simulink model "HGvwab"  (R2020b)
settings: Solver=VariableStepAuto  StartTime=0.0  StopTime=T  MaxStep=MaxStep  RelTol=RelTol  EnableMultiTasking=on
values from neighbouring files (symbols this model uses):
  c = -55    [main.m]
  d = 4    [main.m]
  delay_m = 0    [main.m]
  Iext = 10    [main.m]
  J = 10    [main.m]
  ll = 4    [main.m]
  rule = 1    [main.m]
  T = 30    [main.m]
  x0 = [-55;-6;a;b]    [main.m]
  zHat0 = compute_z(xHat0,Iext)    [main.m]
undefined symbols (not defined in the file or in its folder): C_syst, compute_cond_inv, compute_cond_inv_z, compute_x, compute_z, D_syst, f_syst, g_syst
libraries: simulink x6
settings Model: Creator=pmbernar  LastModifiedBy=Pauline
settings DataIOCC: LimitDataPoints=on  ReturnWorkspaceOutputs=off
settings OptimizationCC: LifeSpan=inf
settings DebuggingCC: AllowSymbolicDim=off  PregeneratedLibrarySubsystemCodeDiagnostic=none  SFUnexpectedBacktrackingDiag=warning  SFNoUnconditionalDefaultTransitionDiag=warning  SFExecutionAtInitializationDiag=none  ArithmeticOperatorsInVariantConditions=warning
settings ModelReferenceCC: PropagateSignalLabelsOutOfModel=off
settings SFSimCC: SimUseLocalCustomCode=off  CustomCodeUndefinedFunction=UseInterfaceOnly
settings RTWCC: RTWUseLocalCustomCode=off
settings CodeAppCC: StateflowObjectComments=on
settings GRTTargetCC: TargetLangStandard=C89/C90 (ANSI)
settings ConfigComp: CovMetricSettings=dw  CovSaveCumulativeToWorkspaceVar=on  CovSaveSingleToWorkspaceVar=on  CovExternalEMLEnable=off

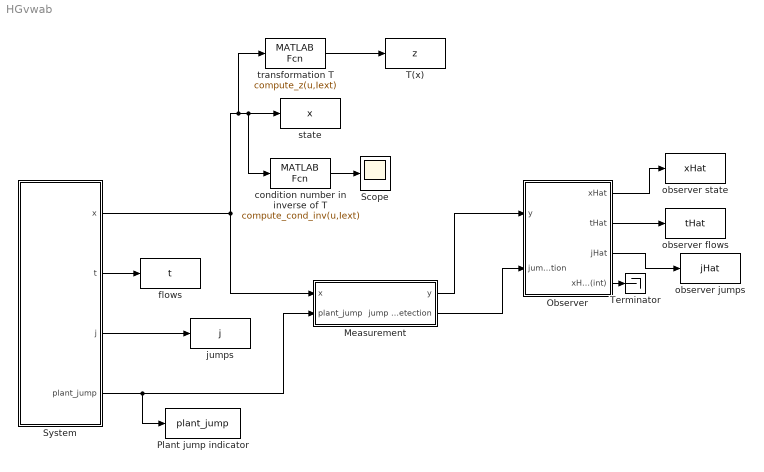
== system HGvwab ==
  Measurement : Subsystem  TreatAsAtomicUnit=on
  Observer : Subsystem  LoadFcn=set_param(gcb,'LinkStatus','none')
      settings: CopyFcn=|
      | set_param(gcb,'LinkStatus','none'),
      | set_param(gcs, 'MaxStep', 'MaxStep', 'RelTol', 'RelTol','Stop time', 'T')
  Plant jump indicator : ToWorkspace  VariableName=plant_jump  SampleTime=-1
  Scope : Scope
  System : Subsystem  LoadFcn=set_param(gcb,'LinkStatus','none')
      settings: CopyFcn=set_param(gcb,'LinkStatus','none')
      mask Display:
      | %image(imread('Hcalneg.jpg'))
      | %plot([5 20 20 5 5],[5 5 20 20 5])
      | %text(8,13,'HyEq_mdl')
      | color('white')
      | port_label('output', 1, 'x')
      | port_label('output', 2, 't')
      | port_label('output', 3, 'j')
  "T(x) " : ToWorkspace  VariableName=z  SampleTime=-1
  Terminator : Terminator
  "condition number in inverse of T " : MATLABFcn  MATLABFcn=compute_cond_inv(u,Iext)
  flows : ToWorkspace  VariableName=t  SampleTime=-1
  jumps : ToWorkspace  VariableName=j  SampleTime=-1
  observer flows : ToWorkspace  VariableName=tHat  SampleTime=-1
  observer jumps : ToWorkspace  VariableName=jHat  SampleTime=-1
  observer state : ToWorkspace  VariableName=xHat  SampleTime=-1
  state : ToWorkspace  VariableName=x  SampleTime=-1
  transformation T : MATLABFcn  MATLABFcn=compute_z(u,Iext)
  wires:
  System/2(t) -> flows/1
  System/3(j) -> jumps/1
  Measurement/1(y) -> Observer/1(y)
  Observer/1(xHat) -> observer state/1
  Observer/2(tHat) -> observer flows/1
  Observer/3(jHat) -> observer jumps/1
  System/1(x) -> Measurement/1(x), transformation T/1, "condition number in inverse of T "/1, state/1
  transformation T/1 -> "T(x) "/1
  "condition number in inverse of T "/1 -> Scope/1
  Observer/4(xHat-(int)) -> Terminator/1
  System/4(plant_jump) -> Plant jump indicator/1, Measurement/2(plant_jump)
  Measurement/2(" jump detection") -> Observer/2(jump detection)

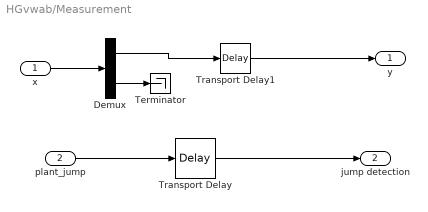
== system HGvwab/Measurement ==
  x : Inport
  plant_jump : Inport  Port=2
  Demux : Demux  Outputs=2
  Terminator : Terminator
  Transport Delay : TransportDelay  DelayTime=delay_m
  Transport Delay1 : TransportDelay  DelayTime=delay_m  InitialOutput=delay_m
  y : Outport  VectorParamsAs1DForOutWhenUnconnected=off
  " jump detection" : Outport  Port=2  VectorParamsAs1DForOutWhenUnconnected=off
  wires:
  x/1 -> Demux/1
  Transport Delay1/1 -> y/1
  Demux/1 -> Transport Delay1/1
  Demux/2 -> Terminator/1
  plant_jump/1 -> Transport Delay/1
  Transport Delay/1 -> " jump detection"/1

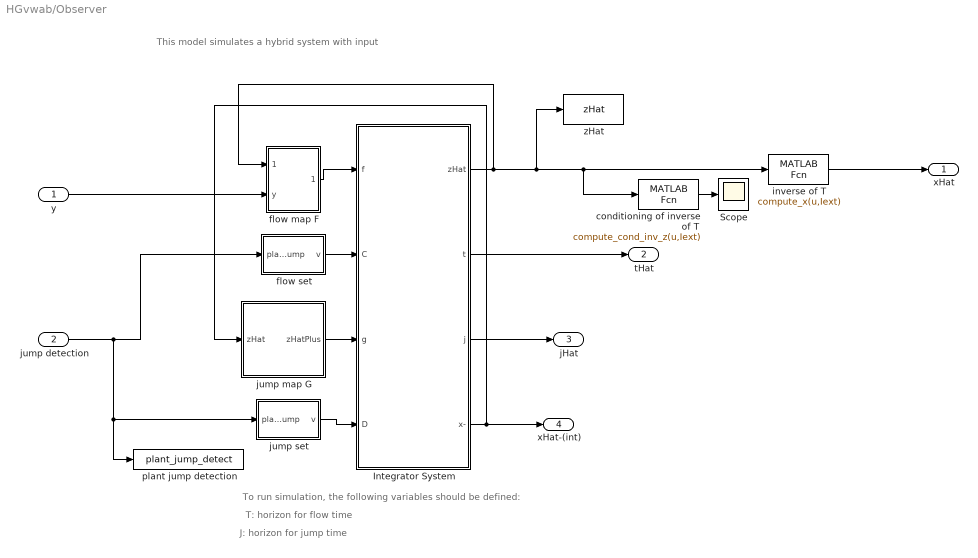
== system HGvwab/Observer ==
  note: J: horizon for jump time
  note: T: horizon for flow time
  note: To run simulation, the following variables should be defined:
  note: This model simulates a hybrid system with input
  y : Inport
  jump detection : Inport  Port=2
  Integrator System : Subsystem  Priority=2  mask(Hybrid Integrator){T=T, J=J, x0=zHat0}
      mask prompts: T "Flow Horizon"; J "Jump Horizon"; x0 "Initial Condition"
      mask help:
      | This block integrates the state of the hybrid system defined by the flow map f (first input), the flow set C (second input), the jump map g (third input) and the jump set D (fourth input).
      | Starting from the initial condition x0 (last mask parameter), the system's state x evolves continuously within the set C, according to f(x,u), but is also subject to jumps within D, according to g(x,u).
      | The block also stops the simulation when the time t is greater than the flow horizon T (first mask parameter), or when the number of jumps j is greater than the jump horizon J (second mask parameter).
      | The outputs of the blocks are respectively x(t), t, j, x(t-).
      mask Help:
      | This block integrates the state of the hybrid system defined by the flow map f (first input), the flow set C (second input), the jump map g (third input) and the jump set D (fourth input).
      | <br>
      | Starting from the initial condition x0 (last mask parameter), the system's state x evolves continuously within the set C, according to f(x,u), but is also subject to jumps within D, according to g(x,u).
      | <br>
      | The block also stops the simulation when the time t is greater than the flow horizon T (first mask parameter), or when the number of jumps j is greater than the jump horizon J (second mask parameter).
      | <br>
      | The outputs of the blocks are respectively x(t), t, j, x(t-).
      | <br>
      | You can right click on the block and "Look under mask" to see what's inside the block.
      | Finally, refer to the manual (HybridSimulator_vXX.pdf) for more detailed information on how this hybrid simulator works.
  Scope : Scope
  conditioning of inverse of T : MATLABFcn  MATLABFcn=compute_cond_inv_z(u,Iext)
  flow map F : MATLAB Function  TreatAsAtomicUnit=on
  "flow set " : MATLAB Function  TreatAsAtomicUnit=on
  inverse of T : MATLABFcn  MATLABFcn=compute_x(u,Iext)
  jump map G : MATLAB Function  Priority=2  TreatAsAtomicUnit=on
  "jump set " : MATLAB Function  TreatAsAtomicUnit=on
  plant jump detection : ToWorkspace  VariableName=plant_jump_detect  SampleTime=-1
  zHat : ToWorkspace  VariableName=zHat  SampleTime=-1
  xHat : Outport  VectorParamsAs1DForOutWhenUnconnected=off
  tHat : Outport  Port=2  VectorParamsAs1DForOutWhenUnconnected=off
  jHat : Outport  Port=3  VectorParamsAs1DForOutWhenUnconnected=off
  xHat-(int) : Outport  Port=4  VectorParamsAs1DForOutWhenUnconnected=off
  wires:
  jump map G/1(zHatPlus) -> Integrator System/3(g)
  "jump set "/1(v) -> Integrator System/4(D)
  y/1 -> flow map F/2(y)
  Integrator System/3(j) -> jHat/1
  Integrator System/2(t) -> tHat/1
  "flow set "/1(v) -> Integrator System/2(C)
  Integrator System/1(zHat) -> zHat/1, conditioning of inverse of T/1, inverse of T/1, flow map F/1(zHat)
  Integrator System/4(x-) -> jump map G/1(zHat), xHat-(int)/1
  flow map F/1(zHatdot) -> Integrator System/1(f)
  inverse of T/1 -> xHat/1
  conditioning of inverse of T/1 -> Scope/1
  jump detection/1 -> "flow set "/1(plant_jump), "jump set "/1(plant_jump), plant jump detection/1

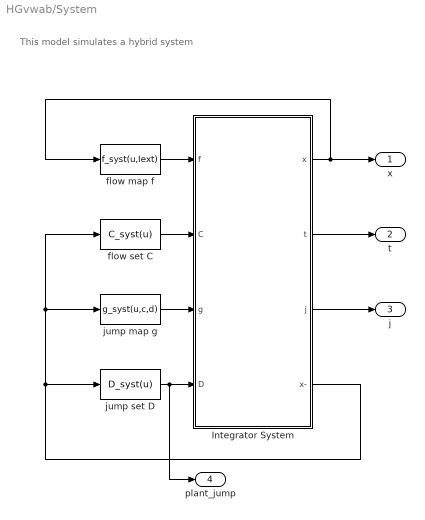
== system HGvwab/System ==
  note: This model simulates a hybrid system
  Integrator System : Subsystem  Priority=2  mask(Hybrid Integrator){T=T, J=J, x0=x0}
      mask prompts: T "Flow Horizon"; J "Jump Horizon"; x0 "Initial Condition"
      mask help:
      | This block integrates the state of the hybrid system defined by the flow map f (first input), the flow set C (second input), the jump map g (third input) and the jump set D (fourth input).
      | Starting from the initial condition x0 (last mask parameter), the system's state x evolves continuously within the set C, according to f(x,u), but is also subject to jumps within D, according to g(x,u).
      | The block also stops the simulation when the time t is greater than the flow horizon T (first mask parameter), or when the number of jumps j is greater than the jump horizon J (second mask parameter).
      | The outputs of the blocks are respectively x(t), t, j, x(t-).
      mask Help:
      | This block integrates the state of the hybrid system defined by the flow map f (first input), the flow set C (second input), the jump map g (third input) and the jump set D (fourth input).
      | <br>
      | Starting from the initial condition x0 (last mask parameter), the system's state x evolves continuously within the set C, according to f(x,u), but is also subject to jumps within D, according to g(x,u).
      | <br>
      | The block also stops the simulation when the time t is greater than the flow horizon T (first mask parameter), or when the number of jumps j is greater than the jump horizon J (second mask parameter).
      | <br>
      | The outputs of the blocks are respectively x(t), t, j, x(t-).
      | <br>
      | You can right click on the block and "Look under mask" to see what's inside the block.
      | Finally, refer to the manual (HybridSimulator_vXX.pdf) for more detailed information on how this hybrid simulator works.
  flow map f : MATLABFcn  MATLABFcn=f_syst(u,Iext)
  flow set C : MATLABFcn  MATLABFcn=C_syst(u)
  jump map g : MATLABFcn  MATLABFcn=g_syst(u,c,d)
  jump set D : MATLABFcn  MATLABFcn=D_syst(u)
  x : Outport  VectorParamsAs1DForOutWhenUnconnected=off
  t : Outport  Port=2  VectorParamsAs1DForOutWhenUnconnected=off
  j : Outport  Port=3  VectorParamsAs1DForOutWhenUnconnected=off
  plant_jump : Outport  Port=4
  wires:
  jump map g/1 -> Integrator System/3(g)
  jump set D/1 -> plant_jump/1, Integrator System/4(D)
  Integrator System/3(j) -> j/1
  Integrator System/2(t) -> t/1
  flow set C/1 -> Integrator System/2(C)
  Integrator System/1(x) -> flow map f/1, x/1
  Integrator System/4(x-) -> flow set C/1, jump map g/1, jump set D/1
  flow map f/1 -> Integrator System/1(f)

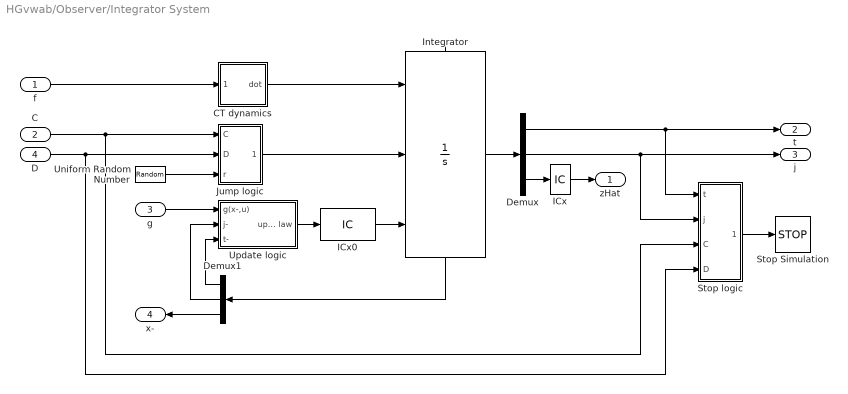
== system HGvwab/Observer/Integrator System ==
  f : Inport
  C : Inport  Port=2
  g : Inport  Port=3
  D : Inport  Port=4
  CT dynamics : Subsystem
  Demux : Demux  Outputs=[1 1 -1]
  Demux1 : Demux  Outputs=[1 1 -1]
  ICx : InitialCondition  Value=x0
  ICx0 : InitialCondition  Value=[0; 0; x0(:)]
  Integrator : Integrator  ExternalReset=level hold  InitialConditionSource=external  ShowStatePort=on  ZeroCross=off
  Jump logic : Subsystem
  Stop Simulation : Stop
  Stop logic : Subsystem
  Uniform Random Number : UniformRandomNumber  Minimum=0  Seed=abs(floor(100*rand))  SampleTime=0
  Update logic : Subsystem
  zHat : Outport  VectorParamsAs1DForOutWhenUnconnected=off
  t : Outport  Port=2  VectorParamsAs1DForOutWhenUnconnected=off
  j : Outport  Port=3  VectorParamsAs1DForOutWhenUnconnected=off
  x- : Outport  Port=4  VectorParamsAs1DForOutWhenUnconnected=off
  wires:
  ICx0/1 -> Integrator/3
  ICx/1 -> zHat/1
  Demux/3 -> ICx/1
  Integrator/State -> Demux1/1
  Demux/2 -> j/1, Stop logic/2(j)
  Demux/1 -> t/1, Stop logic/1(t)
  Update logic/1(update law) -> ICx0/1
  CT dynamics/1(dot) -> Integrator/1
  Stop logic/1(stop) -> Stop Simulation/1
  Integrator/1 -> Demux/1
  C/1 -> Stop logic/3(C), Jump logic/1(C)
  D/1 -> Stop logic/4(D), Jump logic/2(D)
  f/1 -> CT dynamics/1(f(x,u))
  Demux1/3 -> x-/1
  Jump logic/1(jump) -> Integrator/2
  Uniform Random Number/1 -> Jump logic/3(r)
  g/1 -> Update logic/1(g(x-,u))
  Demux1/1 -> Update logic/3(t-)
  Demux1/2 -> Update logic/2(j-)

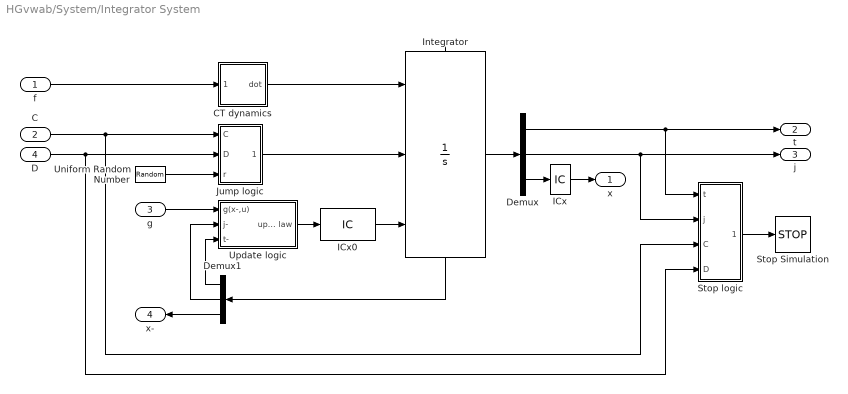
== system HGvwab/System/Integrator System ==
  f : Inport
  C : Inport  Port=2
  g : Inport  Port=3
  D : Inport  Port=4
  CT dynamics : Subsystem
  Demux : Demux  Outputs=[1 1 -1]
  Demux1 : Demux  Outputs=[1 1 -1]
  ICx : InitialCondition  Value=x0
  ICx0 : InitialCondition  Value=[0; 0; x0(:)]
  Integrator : Integrator  ExternalReset=level hold  InitialConditionSource=external  ShowStatePort=on  ZeroCross=off
  Jump logic : Subsystem
  Stop Simulation : Stop
  Stop logic : Subsystem
  Uniform Random Number : UniformRandomNumber  Minimum=0  Seed=abs(floor(100*rand))  SampleTime=0
  Update logic : Subsystem
  x : Outport  VectorParamsAs1DForOutWhenUnconnected=off
  t : Outport  Port=2  VectorParamsAs1DForOutWhenUnconnected=off
  j : Outport  Port=3  VectorParamsAs1DForOutWhenUnconnected=off
  x- : Outport  Port=4  VectorParamsAs1DForOutWhenUnconnected=off
  wires:
  ICx0/1 -> Integrator/3
  ICx/1 -> x/1
  Demux/3 -> ICx/1
  Integrator/State -> Demux1/1
  Demux/2 -> j/1, Stop logic/2(j)
  Demux/1 -> t/1, Stop logic/1(t)
  Update logic/1(update law) -> ICx0/1
  CT dynamics/1(dot) -> Integrator/1
  Stop logic/1(stop) -> Stop Simulation/1
  Integrator/1 -> Demux/1
  C/1 -> Stop logic/3(C), Jump logic/1(C)
  D/1 -> Stop logic/4(D), Jump logic/2(D)
  f/1 -> CT dynamics/1(f(x,u))
  Demux1/3 -> x-/1
  Jump logic/1(jump) -> Integrator/2
  Uniform Random Number/1 -> Jump logic/3(r)
  g/1 -> Update logic/1(g(x-,u))
  Demux1/1 -> Update logic/3(t-)
  Demux1/2 -> Update logic/2(j-)

== system HGvwab/Observer/Integrator System/CT dynamics ==
  f(x,u) : Inport
  Flows : Constant
  Jumps : Constant  Value=0
  Mux : Mux  Inputs=[1 1 -1]
  dot : Outport  VectorParamsAs1DForOutWhenUnconnected=off
  wires:
  Jumps/1 -> Mux/2
  Flows/1 -> Mux/1
  Mux/1 -> dot/1
  f(x,u)/1 -> Mux/3

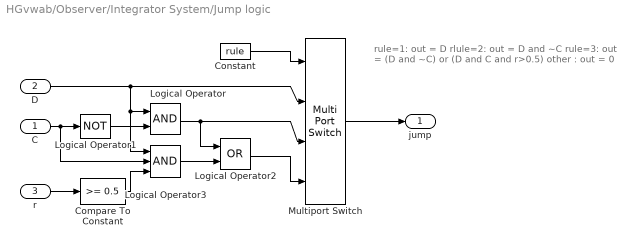
== system HGvwab/Observer/Integrator System/Jump logic ==
  note: rule=1:  out = D
      | rlule=2: out = D and ~C
      | rule=3:  out = (D and ~C)  or (D and C and r>0.5)
      | other :  out = 0
  C : Inport
  D : Inport  Port=2
  r : Inport  Port=3
  Compare To Constant : simulink/Logic and Bit Operations/Compare To Constant  relop=>=  const=0.5  OutDataTypeStr=uint8
  Constant : Constant  Value=rule
  Logical Operator : Logic  AllPortsSameDT=off  OutDataTypeStr=boolean
  Logical Operator1 : Logic  Operator=NOT  Inputs=1  AllPortsSameDT=off  OutDataTypeStr=boolean
  Logical Operator2 : Logic  Operator=OR  AllPortsSameDT=off  OutDataTypeStr=boolean
  Logical Operator3 : Logic  Inputs=3  AllPortsSameDT=off  OutDataTypeStr=boolean
  Multiport Switch : MultiPortSwitch
  jump : Outport  VectorParamsAs1DForOutWhenUnconnected=off
  wires:
  Constant/1 -> Multiport Switch/1
  D/1 -> Logical Operator3/1, Logical Operator/1, Multiport Switch/2
  r/1 -> Compare To Constant/1
  C/1 -> Logical Operator3/2, Logical Operator1/1
  Logical Operator1/1 -> Logical Operator/2
  Logical Operator/1 -> Multiport Switch/3, Logical Operator2/1
  Logical Operator2/1 -> Multiport Switch/4
  Multiport Switch/1 -> jump/1
  Compare To Constant/1 -> Logical Operator3/3
  Logical Operator3/1 -> Logical Operator2/2

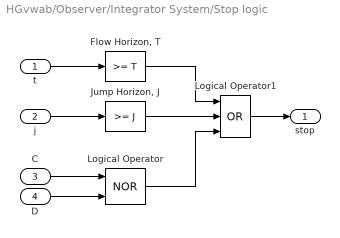
== system HGvwab/Observer/Integrator System/Stop logic ==
  t : Inport
  j : Inport  Port=2
  C : Inport  Port=3
  D : Inport  Port=4
  "Flow Horizon, T" : simulink/Logic and Bit Operations/Compare To Constant  relop=>=  const=T  OutDataTypeStr=uint8  ZeroCross=off
  "Jump Horizon, J" : simulink/Logic and Bit Operations/Compare To Constant  relop=>=  const=J  OutDataTypeStr=uint8  ZeroCross=off
  Logical Operator : Logic  Operator=NOR  AllPortsSameDT=off  OutDataTypeStr=boolean
  Logical Operator1 : Logic  Operator=OR  Inputs=3  AllPortsSameDT=off  OutDataTypeStr=boolean
  stop : Outport  VectorParamsAs1DForOutWhenUnconnected=off
  wires:
  "Flow Horizon, T"/1 -> Logical Operator1/1
  "Jump Horizon, J"/1 -> Logical Operator1/2
  Logical Operator/1 -> Logical Operator1/3
  D/1 -> Logical Operator/2
  t/1 -> "Flow Horizon, T"/1
  j/1 -> "Jump Horizon, J"/1
  C/1 -> Logical Operator/1
  Logical Operator1/1 -> stop/1

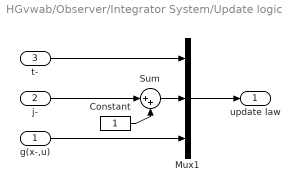
== system HGvwab/Observer/Integrator System/Update logic ==
  g(x-,u) : Inport
  j- : Inport  Port=2
  t- : Inport  Port=3
  Constant : Constant
  Mux1 : Mux  Inputs=[1 1 -1]
  Sum : Sum  Inputs=|++
  update law : Outport  VectorParamsAs1DForOutWhenUnconnected=off
  wires:
  Sum/1 -> Mux1/2
  Mux1/1 -> update law/1
  j-/1 -> Sum/1
  g(x-,u)/1 -> Mux1/3
  t-/1 -> Mux1/1
  Constant/1 -> Sum/2

== system HGvwab/System/Integrator System/CT dynamics ==
  f(x,u) : Inport
  Flows : Constant
  Jumps : Constant  Value=0
  Mux : Mux  Inputs=[1 1 -1]
  dot : Outport  VectorParamsAs1DForOutWhenUnconnected=off
  wires:
  Jumps/1 -> Mux/2
  Flows/1 -> Mux/1
  Mux/1 -> dot/1
  f(x,u)/1 -> Mux/3

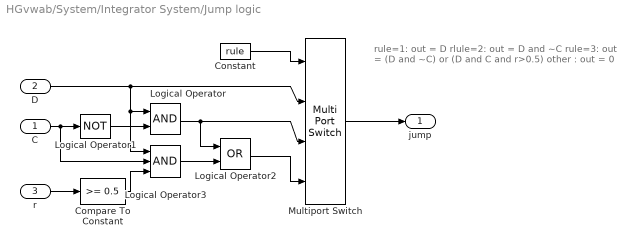
== system HGvwab/System/Integrator System/Jump logic ==
  note: rule=1:  out = D
      | rlule=2: out = D and ~C
      | rule=3:  out = (D and ~C)  or (D and C and r>0.5)
      | other :  out = 0
  C : Inport
  D : Inport  Port=2
  r : Inport  Port=3
  Compare To Constant : simulink/Logic and Bit Operations/Compare To Constant  relop=>=  const=0.5  OutDataTypeStr=uint8
  Constant : Constant  Value=rule
  Logical Operator : Logic  AllPortsSameDT=off  OutDataTypeStr=boolean
  Logical Operator1 : Logic  Operator=NOT  Inputs=1  AllPortsSameDT=off  OutDataTypeStr=boolean
  Logical Operator2 : Logic  Operator=OR  AllPortsSameDT=off  OutDataTypeStr=boolean
  Logical Operator3 : Logic  Inputs=3  AllPortsSameDT=off  OutDataTypeStr=boolean
  Multiport Switch : MultiPortSwitch
  jump : Outport  VectorParamsAs1DForOutWhenUnconnected=off
  wires:
  Constant/1 -> Multiport Switch/1
  D/1 -> Logical Operator3/1, Logical Operator/1, Multiport Switch/2
  r/1 -> Compare To Constant/1
  C/1 -> Logical Operator3/2, Logical Operator1/1
  Logical Operator1/1 -> Logical Operator/2
  Logical Operator/1 -> Multiport Switch/3, Logical Operator2/1
  Logical Operator2/1 -> Multiport Switch/4
  Multiport Switch/1 -> jump/1
  Compare To Constant/1 -> Logical Operator3/3
  Logical Operator3/1 -> Logical Operator2/2

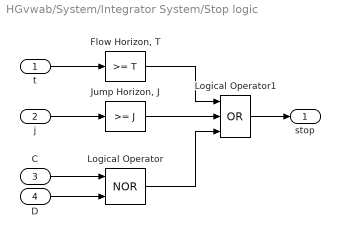
== system HGvwab/System/Integrator System/Stop logic ==
  t : Inport
  j : Inport  Port=2
  C : Inport  Port=3
  D : Inport  Port=4
  "Flow Horizon, T" : simulink/Logic and Bit Operations/Compare To Constant  relop=>=  const=T  OutDataTypeStr=uint8  ZeroCross=off
  "Jump Horizon, J" : simulink/Logic and Bit Operations/Compare To Constant  relop=>=  const=J  OutDataTypeStr=uint8  ZeroCross=off
  Logical Operator : Logic  Operator=NOR  AllPortsSameDT=off  OutDataTypeStr=boolean
  Logical Operator1 : Logic  Operator=OR  Inputs=3  AllPortsSameDT=off  OutDataTypeStr=boolean
  stop : Outport  VectorParamsAs1DForOutWhenUnconnected=off
  wires:
  "Flow Horizon, T"/1 -> Logical Operator1/1
  "Jump Horizon, J"/1 -> Logical Operator1/2
  Logical Operator/1 -> Logical Operator1/3
  D/1 -> Logical Operator/2
  t/1 -> "Flow Horizon, T"/1
  j/1 -> "Jump Horizon, J"/1
  C/1 -> Logical Operator/1
  Logical Operator1/1 -> stop/1

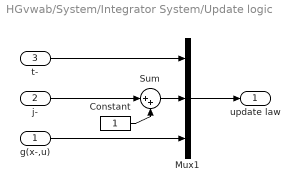
== system HGvwab/System/Integrator System/Update logic ==
  g(x-,u) : Inport
  j- : Inport  Port=2
  t- : Inport  Port=3
  Constant : Constant
  Mux1 : Mux  Inputs=[1 1 -1]
  Sum : Sum  Inputs=|++
  update law : Outport  VectorParamsAs1DForOutWhenUnconnected=off
  wires:
  Sum/1 -> Mux1/2
  Mux1/1 -> update law/1
  j-/1 -> Sum/1
  g(x-,u)/1 -> Mux1/3
  t-/1 -> Mux1/1
  Constant/1 -> Sum/2

== matlab function HGvwab/Observer/flow map F ==
  data: zHat input; zHatdot output; y input; ll parameter; Iext parameter
function zHatdot = F(zHat, y,ll,Iext)

Ac = [0,1,0,0;0,0,1,0;0,0,0,1;0,0,0,0];
Lc = diag([ll;ll^2;ll^3;ll^4]);
K = [3.0777,4.2361,3.0777,1]'; % comes from care(Ac',[1,0,0,0]',eye(4))

x = compute_x(zHat,Iext);

v = x(1);
w = x(2);
a = x(3);
b = x(4);

vdot = 0.04*v^2+5*v+140-w+Iext;
wdot = a*(b*v-w);
vdotdot = (0.04*2*v+5)*vdot-wdot;
wdotdot = a*(b*vdot-wdot);
vdotdotdot = 0.04*2*vdot*vdot+(0.04*2*v+5)*vdotdot-wdotdot;
wdotdotdot = a*(b*vdotdot-wdotdot);

% bounds for saturation |v|<80, |w|<10, |z2|<820 ->  

phi = 0.04*2*2*vdot*vdotdot+0.04*2*vdot*vdotdot+(0.04*2*v+5)*vdotdotdot-wdotdotdot;
phi = min(max(phi,-10^7),10^7);
Bc = [0;0;0;1];

zHatdot = Ac*zHat+Bc*phi+Lc*K*(y(1)-zHat(1));

== matlab function HGvwab/Observer/flow set  ==
  data: plant_jump input; v output
function v  = Chat(plant_jump) 


if (plant_jump== 0)  % flow condition
    v = 1;  % report flow
else
    v = 0;   % do not report flow
end

== matlab function HGvwab/Observer/jump map G ==
  data: zHat input; zHatPlus output; d parameter; Iext parameter; c parameter
function zHatPlus = G(zHat,d,Iext, c)

xHat = compute_x(zHat,Iext);

xHatPlus = [c;xHat(2)+d;xHat(3);xHat(4)];

zHatPlus = compute_z(xHatPlus,Iext);

zHatPlus(1) = min(max(zHatPlus(1),-80),80);
zHatPlus(2) = min(max(zHatPlus(2),-820),820);
zHatPlus(3) = min(max(zHatPlus(3),-820),820);
zHatPlus(4) = min(max(zHatPlus(4),-820),820);

== matlab function HGvwab/Observer/jump set  ==
  data: v output; plant_jump input
function v  = Dhat(plant_jump) 

if (plant_jump > 0)  % jump condition
    v = 1;  % report jump
else
    v = 0;   % do not report jump
end
